simulink model "Copy_of_fast_powertrain"  (R2020b)
settings: Solver=FixedStepAuto  StartTime=0  StopTime=t(end)  RelTol=1e-3
PreLoadFcn:
  | C_sc = 1;
StartFcn:
  | C_sc = 1;
values from neighbouring files (symbols this model uses):
  fc_power_array = [900 900 900 900 900 900 900 900 900 900 900 900 ... (24566 elements, 71x346)]    [fc_power_climb_dp.mat]    (also in fc_power_cruise_dp.mat = [0 0 0 0 0 0 0 0 0 0 0 0 ... (32589 elements, 71x459)]; fc_power_descend_dp.mat = [285.411057245 285.411057245 285.411057245 285.411057245 285; fc_power_takeoff_dp.mat = [0 0 0 0 0 0 0 0 0 0 0 0 ... (23714 elements, 71x334)])
  Ts = old_data.Ts    [model_fc.m]
undefined symbols (not defined in the file or in its folder): DiscIntNeverNeededParam, Ion, Lithium, w
libraries: neural x50, powerlib x30, fuzblock x7, electricdrivelib x2, lib_converters x2, simulink x1
(part 3 of 5)

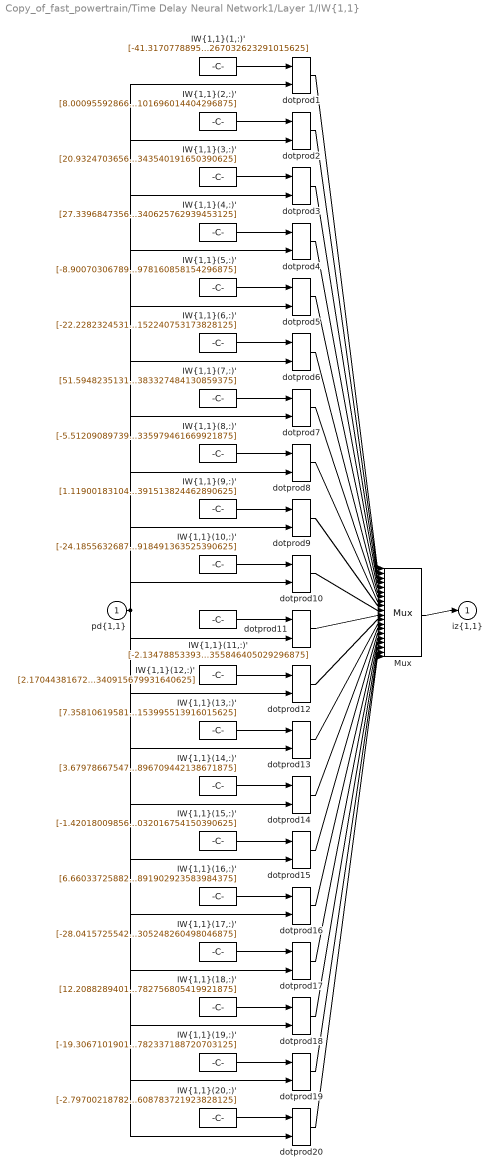
== system Copy_of_fast_powertrain/Time Delay Neural Network1/Layer 1/IW{1,1} ==
  "pd{1,1}" : Inport  PortDimensions=20  SampleTime=0.01
      mask Display: e = 0.06;c1 = [120 230 180]/255;c2 = ([120 230 180]+0)/(256+128);c3 = ([120 230 180]+128)/(256+128);patch([0 1 1 0],[0 0 1 1],c1);patch([0 1 1 1-e 1-e 0+e],[0 0 1 1-e 0+e 0+e],c2);patch([0 0 1 1-e 0+e 0+e],[0 1 1 1-e 1-e 0+e],c3);plot([0 1 1 0 0],[0 0 1 1 0]);
  "IW{1,1}(1,:)'" : Constant  Value=[-41.3170778895787549345186562277376651763916015625;-24.0887056388310867305335705168545246124267578125;-13.8798772268015415676245538634248077869415283203125;-11.567409242390937151867547072470188140869140625;-7.356579925855793788969094748608767986297607421875;4.9515916542348659135086563765071332454681396484375;14.3524439434296144924019245081581175327301025390625;16.54972712574036819432876654900610446929931640625;14.0243285040616729730800216202624142169952392578125;8.05588338287137872839593910612165927886962890625;0.244736738010354282213398846579366363584995269775390625;-6.6453737162459614040699307224713265895843505859375;-8.08441524115644227777011110447347164154052734375;-3.094343005952360226018527100677601993083953857421875;4.26970438586587075491252107894979417324066162109375;3.5510471509297900638557621277868747711181640625;1.931204814168190342371644874219782650470733642578125;5.147881514928489110616283142007887363433837890625;15.346019511090471354464170872233808040618896484375;28.89157804877809354593409807421267032623291015625]
      mask Display: e = 0.06;c1 = [120 150 230]/255;c2 = ([120 150 230]+0)/383;c3 = ([120 150 230]+128)/383;patch([0 1 1 0],[0 0 1 1],c1);patch([0 1 1 1-e 1-e 0+e],[0 0 1 1-e 0+e 0+e],c2);patch([0 0 1 1-e 0+e 0+e],[0 1 1 1-e 1-e 0+e],c3);plot([0 1 1 0 0],[0 0 1 1 0]);disp('Weights');
  "IW{1,1}(10,:)'" : Constant  Value=[-24.185563268711344875327995396219193935394287109375;-17.05035411347990503827531938441097736358642578125;-13.6433375683293132141216119634918868541717529296875;-10.6339863508851077966710363398306071758270263671875;-8.167743630631310480794127215631306171417236328125;-7.68393810138619404170867710490711033344268798828125;-7.310595578676071681911707855761051177978515625;-6.6070230562044311994895906536839902400970458984375;-4.7908556067367129571721307002007961273193359375;-2.130885890521920345008766162209212779998779296875;0.6736905781048412311662332285777665674686431884765625;3.79217370987275526061921482323668897151947021484375;4.9231950163727358216192442341707646846771240234375;6.56156027024927990254354881471954286098480224609375;5.07963430191251763545778885600157082080841064453125;4.58522380417822095211022315197624266147613525390625;4.63238649648575506745373786543495953083038330078125;8.33057908449168138531604199670255184173583984375;16.600928369549830421192382345907390117645263671875;29.7591641296045281706028617918491363525390625]
      mask Display: e = 0.06;c1 = [120 150 230]/255;c2 = ([120 150 230]+0)/383;c3 = ([120 150 230]+128)/383;patch([0 1 1 0],[0 0 1 1],c1);patch([0 1 1 1-e 1-e 0+e],[0 0 1 1-e 0+e 0+e],c2);patch([0 0 1 1-e 0+e 0+e],[0 1 1 1-e 1-e 0+e],c3);plot([0 1 1 0 0],[0 0 1 1 0]);disp('Weights');
  "IW{1,1}(11,:)'" : Constant  Value=[-2.1347885339333476650836018961854279041290283203125;19.6289364994059951641247607767581939697265625;4.14715056300510287456972946529276669025421142578125;1.261358625362304142214497915119864046573638916015625;3.84623883470571126252934845979325473308563232421875;-7.1682582085659962700674441293813288211822509765625;-3.736923646637921425650574747123755514621734619140625;-5.88069141749093748927634806022979319095611572265625;-5.55573602274217481777895955019630491733551025390625;4.31752698833330317285117416759021580219268798828125;-1.1252300459187354331191954770474694669246673583984375;4.05713927249998551616272379760630428791046142578125;1.197702286576397767703383578918874263763427734375;-1.9553589340063435297878413621219806373119354248046875;1.6492618632624937990982516566873528063297271728515625;0.2910930951259309562573207585955969989299774169921875;-7.48533898139895992329684304422698915004730224609375;-5.0718983260841241644811816513538360595703125;-9.951981369443966940480095217935740947723388671875;16.351487277274980414176752674393355846405029296875]
      mask Display: e = 0.06;c1 = [120 150 230]/255;c2 = ([120 150 230]+0)/383;c3 = ([120 150 230]+128)/383;patch([0 1 1 0],[0 0 1 1],c1);patch([0 1 1 1-e 1-e 0+e],[0 0 1 1-e 0+e 0+e],c2);patch([0 0 1 1-e 0+e 0+e],[0 1 1 1-e 1-e 0+e],c3);plot([0 1 1 0 0],[0 0 1 1 0]);disp('Weights');
  "IW{1,1}(12,:)'" : Constant  Value=[2.170443816728891750500451962579973042011260986328125;4.831373528298119168766788789071142673492431640625;3.720585501332140498931266847648657858371734619140625;-0.318133659340753049971084465141757391393184661865234375;-0.475728325064818824419177190065965987741947174072265625;-1.51040958520863544123358224169351160526275634765625;2.69378750685471768377965418039821088314056396484375;-1.96104009447486671291471793665550649166107177734375;-3.015653540352828176906996304751373827457427978515625;0.29681634914598553631748245607013814151287078857421875;-3.39010087809587101759234428755007684230804443359375;-3.109983657771648868362035500467754900455474853515625;-2.5953120035258248066156738786958158016204833984375;2.638838351776431334627659452962689101696014404296875;5.737602587752082428096400690264999866485595703125;2.73716197207968914284492711885832250118255615234375;-1.03884155019751123205651310854591429233551025390625;0.70165190413190947626986826435313560068607330322265625;-6.92628258625202430920353435794822871685028076171875;-5.28110531151323758791704676696099340915679931640625]
      mask Display: e = 0.06;c1 = [120 150 230]/255;c2 = ([120 150 230]+0)/383;c3 = ([120 150 230]+128)/383;patch([0 1 1 0],[0 0 1 1],c1);patch([0 1 1 1-e 1-e 0+e],[0 0 1 1-e 0+e 0+e],c2);patch([0 0 1 1-e 0+e 0+e],[0 1 1 1-e 1-e 0+e],c3);plot([0 1 1 0 0],[0 0 1 1 0]);disp('Weights');
  "IW{1,1}(13,:)'" : Constant  Value=[7.358106195812315064586073276586830615997314453125;1.6831218618925074537173713906668126583099365234375;-2.8683861634367673332235426642000675201416015625;-3.85951595603854524796361147309653460979461669921875;-2.419423126387662659197985703940503299236297607421875;-1.588508626987817251574597321450710296630859375;-1.37264008448260010908370531979016959667205810546875;-1.54854636023814773437834446667693555355072021484375;-0.10374636418391712522346637115333578549325466156005859375;-0.5967477756502417296502471799612976610660552978515625;0.43226922179724536210443375239265151321887969970703125;0.5628800436407732643573353925603441894054412841796875;0.8431480665077806246898717290605418384075164794921875;0.63425152767940617959396831793128512799739837646484375;1.3560400000311558788013144294382072985172271728515625;1.06751403398893529583801864646375179290771484375;-1.1827681419481888003275571463746018707752227783203125;-4.5508660633518918103845862788148224353790283203125;-8.1547629852644458736676824628375470638275146484375;-12.0765016778454796764208367676474153995513916015625]
      mask Display: e = 0.06;c1 = [120 150 230]/255;c2 = ([120 150 230]+0)/383;c3 = ([120 150 230]+128)/383;patch([0 1 1 0],[0 0 1 1],c1);patch([0 1 1 1-e 1-e 0+e],[0 0 1 1-e 0+e 0+e],c2);patch([0 0 1 1-e 0+e 0+e],[0 1 1 1-e 1-e 0+e],c3);plot([0 1 1 0 0],[0 0 1 1 0]);disp('Weights');
  "IW{1,1}(14,:)'" : Constant  Value=[3.67978667547009674620994701399467885494232177734375;-2.22690009056678572818555039702914655208587646484375;-0.79222376523893933697451075204298831522464752197265625;-6.8093908520768895442643042770214378833770751953125;-2.572056436179115390672222929424606263637542724609375;-1.0626538149219673101697480888105928897857666015625;0.5276216253397276734204979220521636307239532470703125;2.0319562855862702832610011682845652103424072265625;4.9281641317842979077568088541738688945770263671875;2.773369998445488260330193952540867030620574951171875;0.96562902640608372362152067580609582364559173583984375;6.66870819884032695057385353720746934413909912109375;4.0853706891057530725674951099790632724761962890625;-3.780792512882989786504595031146891415119171142578125;-7.9357944400793751782430263119749724864959716796875;-6.37633154443981009507069757091812789440155029296875;0.75252557231104411084032790313358418643474578857421875;3.713808685864766090389821329154074192047119140625;3.38778820457910878616303307353518903255462646484375;4.62408844976101374157906320760957896709442138671875]
      mask Display: e = 0.06;c1 = [120 150 230]/255;c2 = ([120 150 230]+0)/383;c3 = ([120 150 230]+128)/383;patch([0 1 1 0],[0 0 1 1],c1);patch([0 1 1 1-e 1-e 0+e],[0 0 1 1-e 0+e 0+e],c2);patch([0 0 1 1-e 0+e 0+e],[0 1 1 1-e 1-e 0+e],c3);plot([0 1 1 0 0],[0 0 1 1 0]);disp('Weights');
  "IW{1,1}(15,:)'" : Constant  Value=[-1.420180098569664206564766573137603700160980224609375;-5.51110982430032692036547814495861530303955078125;-5.20947745625726010842981850146315991878509521484375;-14.6997746442128800481441430747509002685546875;-8.8563278920764787471853196620941162109375;-0.9626373423566885190183484155568294227123260498046875;6.19541237091466800990247065783478319644927978515625;8.8144073732205558968644254491664469242095947265625;12.296059111145755338156959624029695987701416015625;7.9205582139870909230694451252929866313934326171875;3.785811551668564423067664392874576151371002197265625;-5.5243128402192116510605046642012894153594970703125;-10.001006466530355965005583129823207855224609375;-8.889928686249508160699406289495527744293212890625;-3.84096755903057474057504805386997759342193603515625;2.4065504070994290231055856565944850444793701171875;3.914269531419424907880966202355921268463134765625;6.43574838587781972165657862205989658832550048828125;20.02672266276139367846553795970976352691650390625;-8.6135092808080031545614474453032016754150390625]
      mask Display: e = 0.06;c1 = [120 150 230]/255;c2 = ([120 150 230]+0)/383;c3 = ([120 150 230]+128)/383;patch([0 1 1 0],[0 0 1 1],c1);patch([0 1 1 1-e 1-e 0+e],[0 0 1 1-e 0+e 0+e],c2);patch([0 0 1 1-e 0+e 0+e],[0 1 1 1-e 1-e 0+e],c3);plot([0 1 1 0 0],[0 0 1 1 0]);disp('Weights');
  "IW{1,1}(16,:)'" : Constant  Value=[6.6603372588299354362106896587647497653961181640625;-0.8908372930182395510456672127475030720233917236328125;5.327501255420738601742414175532758235931396484375;15.32497122996134208960938849486410617828369140625;10.790263493254013127398138749413192272186279296875;1.0196787390633499370551362517289817333221435546875;-5.69550501395408392824037946411408483982086181640625;-11.3091877191841962968510415521450340747833251953125;-10.578463028595951556098953005857765674591064453125;-9.5307296775407497335663720150478184223175048828125;-2.19973343032226242854676456772722303867340087890625;3.735648738789860257014652233920060098171234130859375;11.079809353653434556008505751378834247589111328125;8.9052404932124584746588880079798400402069091796875;3.4040744108171434589849013718776404857635498046875;-1.225929473324251173238508272334001958370208740234375;-3.28411757385438018985723829246126115322113037109375;-10.3218805156491679753116841311566531658172607421875;-12.8732991153864446687293821014463901519775390625;3.45410954567542116677714147954247891902923583984375]
      mask Display: e = 0.06;c1 = [120 150 230]/255;c2 = ([120 150 230]+0)/383;c3 = ([120 150 230]+128)/383;patch([0 1 1 0],[0 0 1 1],c1);patch([0 1 1 1-e 1-e 0+e],[0 0 1 1-e 0+e 0+e],c2);patch([0 0 1 1-e 0+e 0+e],[0 1 1 1-e 1-e 0+e],c3);plot([0 1 1 0 0],[0 0 1 1 0]);disp('Weights');
  "IW{1,1}(17,:)'" : Constant  Value=[-28.04157255425118222547098412178456783294677734375;-5.3809637724850656326225362136028707027435302734375;5.17695541887508081657642833306454122066497802734375;11.16804148725753975668339990079402923583984375;12.0601664903482248547561539453454315662384033203125;7.36291293894431664313060537097044289112091064453125;5.5119750429278298042845563031733036041259765625;-2.661671141807496088205198248033411800861358642578125;-4.4897286315137865386759585817344486713409423828125;-0.502920581020447343689738772809505462646484375;-0.5422578739548782333912413378129713237285614013671875;-1.716441764453623619601785321719944477081298828125;1.1676228984111858277827877827803604304790496826171875;5.550100097403696253195448662154376506805419921875;7.51119188051158293006892563425935804843902587890625;5.740538523639262535880334326066076755523681640625;1.8215987865340081963694274236331693828105926513671875;-3.41564694209144281700218925834633409976959228515625;-2.506787719899347788299337480566464364528656005859375;-10.8136694568940452398919660481624305248260498046875]
      mask Display: e = 0.06;c1 = [120 150 230]/255;c2 = ([120 150 230]+0)/383;c3 = ([120 150 230]+128)/383;patch([0 1 1 0],[0 0 1 1],c1);patch([0 1 1 1-e 1-e 0+e],[0 0 1 1-e 0+e 0+e],c2);patch([0 0 1 1-e 0+e 0+e],[0 1 1 1-e 1-e 0+e],c3);plot([0 1 1 0 0],[0 0 1 1 0]);disp('Weights');
  "IW{1,1}(18,:)'" : Constant  Value=[12.2088289401585239346559319528751075267791748046875;11.207627170941886873833936988376080989837646484375;8.120166375458776286677675670944154262542724609375;4.45666694105473037978981665219180285930633544921875;-4.4224351247064124237340365652926266193389892578125;-6.20601126716516926506983509170822799205780029296875;-1.9195754434346776751141305794590152800083160400390625;-3.13496102854807379145540835452266037464141845703125;-2.32668178326190489002556205377914011478424072265625;0.670511817366107987226087061571888625621795654296875;0.89232140437771600982586051031830720603466033935546875;0.55752894691838772445180438808165490627288818359375;-3.33344947856499818072961716097779572010040283203125;1.8208920236868164632682010051212273538112640380859375;5.4889024169390694396497565321624279022216796875;1.5847163583448542478748777284636162221431732177734375;-5.3921423981682092829714747495017945766448974609375;-8.405302129591763815597005304880440235137939453125;-8.864741878767407712302883737720549106597900390625;-3.543055787799016087546988273970782756805419921875]
      mask Display: e = 0.06;c1 = [120 150 230]/255;c2 = ([120 150 230]+0)/383;c3 = ([120 150 230]+128)/383;patch([0 1 1 0],[0 0 1 1],c1);patch([0 1 1 1-e 1-e 0+e],[0 0 1 1-e 0+e 0+e],c2);patch([0 0 1 1-e 0+e 0+e],[0 1 1 1-e 1-e 0+e],c3);plot([0 1 1 0 0],[0 0 1 1 0]);disp('Weights');
  "IW{1,1}(19,:)'" : Constant  Value=[-19.30671019010623012945870868861675262451171875;-21.983671689361745649193835561163723468780517578125;-11.103043353793257352890577749349176883697509765625;-0.279565088451577903327915919362567365169525146484375;9.0057348671534942496919029508717358112335205078125;11.408177187217649617423376184888184070587158203125;10.029518245539403409338774508796632289886474609375;4.33827750612211815450791618786752223968505859375;6.97972260717902681648183715878985822200775146484375;8.3558582696726748650917215854860842227935791015625;3.49812962932533455528982813120819628238677978515625;1.094973913609437854432826497941277921199798583984375;0.82543490581334777456135043394169770181179046630859375;-0.68629990853895694868924692855216562747955322265625;0.0468479576123603524973049161417293362319469451904296875;-4.7912054993083206255732875433750450611114501953125;-1.786395953938544334249627354438416659832000732421875;-6.22266231890149068561868261895142495632171630859375;6.907932831061526002258688095025718212127685546875;5.413336757037843227635676157660782337188720703125]
      mask Display: e = 0.06;c1 = [120 150 230]/255;c2 = ([120 150 230]+0)/383;c3 = ([120 150 230]+128)/383;patch([0 1 1 0],[0 0 1 1],c1);patch([0 1 1 1-e 1-e 0+e],[0 0 1 1-e 0+e 0+e],c2);patch([0 0 1 1-e 0+e 0+e],[0 1 1 1-e 1-e 0+e],c3);plot([0 1 1 0 0],[0 0 1 1 0]);disp('Weights');
  "IW{1,1}(2,:)'" : Constant  Value=[8.0009559286644194031623555929400026798248291015625;0.29799913640694886129978158351150341331958770751953125;2.199307294349767349928015391924418509006500244140625;-0.101158104774415169568868577698594890534877777099609375;-3.272729845188205644035406294278800487518310546875;2.52183259058507047711827908642590045928955078125;-1.46306994719022664952490231371484696865081787109375;-0.571724712775646626283787554712034761905670166015625;0.4244111816213844701195512243430130183696746826171875;-2.11138170909325406654488688218407332897186279296875;-0.1092852808671377629057275271406979300081729888916015625;-7.0818638804236986317164337378926575183868408203125;-1.57683215732416659449199869413860142230987548828125;3.46336741857540975075835376628674566745758056640625;4.80213581541669309871167570236138999462127685546875;2.82902758629478956464708971907384693622589111328125;-1.7424597394520520143856856520869769155979156494140625;-3.902954257014578320905684449826367199420928955078125;2.9544813906346103493660848471336066722869873046875;-9.4713163438792360437901152181439101696014404296875]
      mask Display: e = 0.06;c1 = [120 150 230]/255;c2 = ([120 150 230]+0)/383;c3 = ([120 150 230]+128)/383;patch([0 1 1 0],[0 0 1 1],c1);patch([0 1 1 1-e 1-e 0+e],[0 0 1 1-e 0+e 0+e],c2);patch([0 0 1 1-e 0+e 0+e],[0 1 1 1-e 1-e 0+e],c3);plot([0 1 1 0 0],[0 0 1 1 0]);disp('Weights');
  "IW{1,1}(20,:)'" : Constant  Value=[-2.797002187821615137863773270510137081146240234375;-10.31295322399305547378389746882021427154541015625;-1.55660953829066528442126582376658916473388671875;3.35580071000512081269562258967198431491851806640625;5.9643923538503411663214137661270797252655029296875;5.39805766669024933435139246284961700439453125;2.014178251230946958827416892745532095432281494140625;-0.5077485053936430237087051864364184439182281494140625;0.44283688715125801849126219167374074459075927734375;-0.84923676595938868416624245583079755306243896484375;-1.0839363293868820026233379394398070871829986572265625;2.74830351179496457092454875237308442592620849609375;5.96715115443901300551488020573742687702178955078125;10.446421954846481838785621221177279949188232421875;9.2391410777889628747061578906141221523284912109375;3.9956120733058124727676840848289430141448974609375;-2.73014654632758801966474493383429944515228271484375;-4.92810777807717403931064836797304451465606689453125;-6.188792555902221437236221390776336193084716796875;-14.4144108890875362050110197742469608783721923828125]
      mask Display: e = 0.06;c1 = [120 150 230]/255;c2 = ([120 150 230]+0)/383;c3 = ([120 150 230]+128)/383;patch([0 1 1 0],[0 0 1 1],c1);patch([0 1 1 1-e 1-e 0+e],[0 0 1 1-e 0+e 0+e],c2);patch([0 0 1 1-e 0+e 0+e],[0 1 1 1-e 1-e 0+e],c3);plot([0 1 1 0 0],[0 0 1 1 0]);disp('Weights');
  "IW{1,1}(3,:)'" : Constant  Value=[20.932470365689123781294256332330405712127685546875;18.254007786078663144735401147045195102691650390625;11.545421494161882236539895529858767986297607421875;-0.4887756653028054731890961193130351603031158447265625;-8.76398413124098851767485029995441436767578125;-12.57365231422826212792642763815820217132568359375;-7.46222359613562158386912415153346955776214599609375;-4.808412478315300830900014261715114116668701171875;-6.0961149428762926305580549524165689945220947265625;-7.3019081107598680091541609726846218109130859375;-3.070212599719938761921866898774169385433197021484375;-1.3184986949957842039538036260637454688549041748046875;-1.2993064234001974188714711999637074768543243408203125;0.406971975746562630860125864273868501186370849609375;-1.0449934646656526826546951269847340881824493408203125;6.169523300947691524243055027909576892852783203125;1.81080629847727525572054219082929193973541259765625;5.59354256645015102122897587832994759082794189453125;-1.485107007839122861270197972771711647510528564453125;-10.7319771586214418590543573372997343540191650390625]
      mask Display: e = 0.06;c1 = [120 150 230]/255;c2 = ([120 150 230]+0)/383;c3 = ([120 150 230]+128)/383;patch([0 1 1 0],[0 0 1 1],c1);patch([0 1 1 1-e 1-e 0+e],[0 0 1 1-e 0+e 0+e],c2);patch([0 0 1 1-e 0+e 0+e],[0 1 1 1-e 1-e 0+e],c3);plot([0 1 1 0 0],[0 0 1 1 0]);disp('Weights');
  "IW{1,1}(4,:)'" : Constant  Value=[27.339684735619670163941918872296810150146484375;8.496357856765598626225255429744720458984375;-6.362755084862403265333341551013290882110595703125;-12.7773678444801674913833267055451869964599609375;-10.492634466608620869010337628424167633056640625;-9.67105286856625667724074446596205234527587890625;-3.440768679224401438432323629967868328094482421875;0.2963145832070235297095450732740573585033416748046875;5.7437713069473463889380582259036600589752197265625;0.3476258632510009771721115612308494746685028076171875;0.552428702577281161012479060445912182331085205078125;3.393992684218976929599875802523456513881683349609375;-1.6843270831895862382765471920720301568508148193359375;-6.6691540021836797080823089345358312129974365234375;-7.6569929153395168697215922293253242969512939453125;-4.88877927553946367567050401703454554080963134765625;-0.78681722837249612467758197453804314136505126953125;-0.0568690636677235961116139151272363960742950439453125;6.4993261608193648726228275336325168609619140625;8.56317161450824215762622770853340625762939453125]
      mask Display: e = 0.06;c1 = [120 150 230]/255;c2 = ([120 150 230]+0)/383;c3 = ([120 150 230]+128)/383;patch([0 1 1 0],[0 0 1 1],c1);patch([0 1 1 1-e 1-e 0+e],[0 0 1 1-e 0+e 0+e],c2);patch([0 0 1 1-e 0+e 0+e],[0 1 1 1-e 1-e 0+e],c3);plot([0 1 1 0 0],[0 0 1 1 0]);disp('Weights');
  "IW{1,1}(5,:)'" : Constant  Value=[-8.9007030678935148415575895342044532299041748046875;9.4651280143608769179763839929364621639251708984375;2.459275957901349674017410507076419889926910400390625;3.7583207043845927586289690225385129451751708984375;1.82154654944120775184046578942798078060150146484375;1.421627956337805809283736380166374146938323974609375;-0.7058342521599818564226325179333798587322235107421875;-2.992863439742887265992976608686149120330810546875;-5.2068906654741358153160035726614296436309814453125;-1.66773704253629428961858138791285455226898193359375;-1.9184820671787401469288170119398273527622222900390625;-5.189770753495704269653288065455853939056396484375;-3.424954548731278247686304894159547984600067138671875;3.79075968895624715315761932288296520709991455078125;7.4365298630443561478386982344090938568115234375;6.32941151198017326606759525020606815814971923828125;-1.2726758449697410657819318657857365906238555908203125;-5.25567297078029493917483705445192754268646240234375;-2.26274858455408978130662944749929010868072509765625;-4.2604163572358100253723023342899978160858154296875]
      mask Display: e = 0.06;c1 = [120 150 230]/255;c2 = ([120 150 230]+0)/383;c3 = ([120 150 230]+128)/383;patch([0 1 1 0],[0 0 1 1],c1);patch([0 1 1 1-e 1-e 0+e],[0 0 1 1-e 0+e 0+e],c2);patch([0 0 1 1-e 0+e 0+e],[0 1 1 1-e 1-e 0+e],c3);plot([0 1 1 0 0],[0 0 1 1 0]);disp('Weights');
  "IW{1,1}(6,:)'" : Constant  Value=[-22.22823245318267026959802024066448211669921875;-2.61267557073272627121696132235229015350341796875;-6.09690996180808664206551839015446603298187255859375;0.5252305434929851468695005678455345332622528076171875;5.18797140766390985078260200680233538150787353515625;1.020876156381517407822911991388536989688873291015625;8.70257213333764667595460196025669574737548828125;5.2204624128180956432743187178857624530792236328125;-0.8366628262687212380654955268255434930324554443359375;-0.373197414506467595174399320967495441436767578125;-6.92678541912431366966984569444321095943450927734375;0.10324869827143635936383958551232353784143924713134765625;1.2418435739121991279176882017054595053195953369140625;1.0557948454136596438956985366530716419219970703125;3.01402759675961018359657828113995492458343505859375;4.22146805757340981557490522391162812709808349609375;7.247146300064496671211600187234580516815185546875;4.3041061071129007586932857520878314971923828125;-9.6874140400343602408383958390913903713226318359375;-3.2759926367543688030536941369064152240753173828125]
      mask Display: e = 0.06;c1 = [120 150 230]/255;c2 = ([120 150 230]+0)/383;c3 = ([120 150 230]+128)/383;patch([0 1 1 0],[0 0 1 1],c1);patch([0 1 1 1-e 1-e 0+e],[0 0 1 1-e 0+e 0+e],c2);patch([0 0 1 1-e 0+e 0+e],[0 1 1 1-e 1-e 0+e],c3);plot([0 1 1 0 0],[0 0 1 1 0]);disp('Weights');
  "IW{1,1}(7,:)'" : Constant  Value=[51.5948235131668724307019147090613842010498046875;18.479203641606357422233486431650817394256591796875;-0.1138401529098100883885535949957557022571563720703125;-6.98963796653444280337907912326045334339141845703125;-11.170389097549676904463922255672514438629150390625;-10.4819913877186223771786899305880069732666015625;-9.247598137383402416844546678476035594940185546875;-7.17700869258198981270879812655039131641387939453125;-2.6320741480940785805842097033746540546417236328125;-2.602296546208933580857092238147743046283721923828125;0.2042727877142753722949919392704032361507415771484375;3.9466909235221550034111714921891689300537109375;2.978154313847202416809523128904402256011962890625;-0.2970520106042477959107372953440062701702117919921875;-4.93554185989632543396510300226509571075439453125;-8.604976836124681227602195576764643192291259765625;-8.068677822123898835116051486693322658538818359375;-8.78376927972495735730262822471559047698974609375;0.47388675040789696168985756230540573596954345703125;16.67770704955804461633306345902383327484130859375]
      mask Display: e = 0.06;c1 = [120 150 230]/255;c2 = ([120 150 230]+0)/383;c3 = ([120 150 230]+128)/383;patch([0 1 1 0],[0 0 1 1],c1);patch([0 1 1 1-e 1-e 0+e],[0 0 1 1-e 0+e 0+e],c2);patch([0 0 1 1-e 0+e 0+e],[0 1 1 1-e 1-e 0+e],c3);plot([0 1 1 0 0],[0 0 1 1 0]);disp('Weights');
  "IW{1,1}(8,:)'" : Constant  Value=[-5.5120908973902178473736057640053331851959228515625;-0.08857216638173925904453653856762684881687164306640625;-6.8524858480580181918639937066473066806793212890625;-4.2453872729833204147098513203673064708709716796875;-1.7177497627532272161943183164112269878387451171875;4.06465131407648794237275069463066756725311279296875;5.13777173224305361287633786560036242008209228515625;3.56461861949192293508303919224999845027923583984375;-0.453789369166626543883324984562932513654232025146484375;-0.56670916479507804641713164528482593595981597900390625;-4.24873351646846497686738075572066009044647216796875;2.640255431642579697637529534404166042804718017578125;-1.24500832619264745204645805642940104007720947265625;1.492862977137506153013646326144225895404815673828125;1.0004088100251049553435223060660064220428466796875;2.33866054122455846453476624446921050548553466796875;5.0613013830595861008987412787973880767822265625;3.733246583413986297017572724143974483013153076171875;-5.1544106155657498646860403823666274547576904296875;-4.80560696182090918426865755463950335979461669921875]
      mask Display: e = 0.06;c1 = [120 150 230]/255;c2 = ([120 150 230]+0)/383;c3 = ([120 150 230]+128)/383;patch([0 1 1 0],[0 0 1 1],c1);patch([0 1 1 1-e 1-e 0+e],[0 0 1 1-e 0+e 0+e],c2);patch([0 0 1 1-e 0+e 0+e],[0 1 1 1-e 1-e 0+e],c3);plot([0 1 1 0 0],[0 0 1 1 0]);disp('Weights');
  "IW{1,1}(9,:)'" : Constant  Value=[1.1190018310491545161511339756543748080730438232421875;-9.99456168542398160070661106146872043609619140625;-6.05258353940696025574652594514191150665283203125;-7.28848460783531582052319208742119371891021728515625;-0.8187356429915058075863498743274249136447906494140625;5.16051913868130096574304843670688569545745849609375;5.9688291019320995900443449500016868114471435546875;2.700108935388829234369723053532652556896209716796875;2.77621122768115125012400312698446214199066162109375;-1.219439809609997649175738843041472136974334716796875;-0.65899091759310446381192605258547700941562652587890625;-2.929613833743692108413370078778825700283050537109375;0.1052108163845257848834080505184829235076904296875;-0.34501059064822758859492068950203247368335723876953125;1.1175172915267108653125660566729493439197540283203125;4.27864428805897745178299373947083950042724609375;5.42493416790487259504516259767115116119384765625;2.13665947942197487208204620401374995708465576171875;-0.259858993996790577085675977286882698535919189453125;-7.78855454396885082957169288420118391513824462890625]
      mask Display: e = 0.06;c1 = [120 150 230]/255;c2 = ([120 150 230]+0)/383;c3 = ([120 150 230]+128)/383;patch([0 1 1 0],[0 0 1 1],c1);patch([0 1 1 1-e 1-e 0+e],[0 0 1 1-e 0+e 0+e],c2);patch([0 0 1 1-e 0+e 0+e],[0 1 1 1-e 1-e 0+e],c3);plot([0 1 1 0 0],[0 0 1 1 0]);disp('Weights');
  Mux : Mux  Inputs=20
      mask Display: e = 0.06;c1 = [120 150 230]/255;c2 = ([120 150 230]+0)/383;c3 = ([120 150 230]+128)/383;patch([0 1 1 0],[0 0 1 1],c1);patch([0 1 1 1-e 1-e 0+e],[0 0 1 1-e 0+e 0+e],c2);patch([0 0 1 1-e 0+e 0+e],[0 1 1 1-e 1-e 0+e],c3);plot([0 1 1 0 0],[0 0 1 1 0]);disp('Mux');
  dotprod{1..20} (20 alike) : neural/Weight Functions/dotprod
  "iz{1,1}" : Outport
      mask Display: e = 0.06;c1 = [120 230 180]/255;c2 = ([120 230 180]+0)/(256+128);c3 = ([120 230 180]+128)/(256+128);patch([0 1 1 0],[0 0 1 1],c1);patch([0 1 1 1-e 1-e 0+e],[0 0 1 1-e 0+e 0+e],c2);patch([0 0 1 1-e 0+e 0+e],[0 1 1 1-e 1-e 0+e],c3);plot([0 1 1 0 0],[0 0 1 1 0]);
  wires:
  Mux/1 -> "iz{1,1}"/1
  dotprod20/1 -> Mux/20
  "IW{1,1}(20,:)'"/1 -> dotprod20/1
  dotprod19/1 -> Mux/19
  "IW{1,1}(19,:)'"/1 -> dotprod19/1
  dotprod18/1 -> Mux/18
  "IW{1,1}(18,:)'"/1 -> dotprod18/1
  dotprod17/1 -> Mux/17
  "IW{1,1}(17,:)'"/1 -> dotprod17/1
  dotprod16/1 -> Mux/16
  "IW{1,1}(16,:)'"/1 -> dotprod16/1
  dotprod15/1 -> Mux/15
  "IW{1,1}(15,:)'"/1 -> dotprod15/1
  dotprod14/1 -> Mux/14
  "IW{1,1}(14,:)'"/1 -> dotprod14/1
  dotprod13/1 -> Mux/13
  "IW{1,1}(13,:)'"/1 -> dotprod13/1
  dotprod12/1 -> Mux/12
  "IW{1,1}(12,:)'"/1 -> dotprod12/1
  dotprod11/1 -> Mux/11
  "IW{1,1}(11,:)'"/1 -> dotprod11/1
  dotprod10/1 -> Mux/10
  "IW{1,1}(10,:)'"/1 -> dotprod10/1
  dotprod9/1 -> Mux/9
  "IW{1,1}(9,:)'"/1 -> dotprod9/1
  dotprod8/1 -> Mux/8
  "IW{1,1}(8,:)'"/1 -> dotprod8/1
  dotprod7/1 -> Mux/7
  "IW{1,1}(7,:)'"/1 -> dotprod7/1
  dotprod6/1 -> Mux/6
  "IW{1,1}(6,:)'"/1 -> dotprod6/1
  dotprod5/1 -> Mux/5
  "IW{1,1}(5,:)'"/1 -> dotprod5/1
  dotprod4/1 -> Mux/4
  "IW{1,1}(4,:)'"/1 -> dotprod4/1
  dotprod3/1 -> Mux/3
  "IW{1,1}(3,:)'"/1 -> dotprod3/1
  dotprod2/1 -> Mux/2
  "IW{1,1}(2,:)'"/1 -> dotprod2/1
  dotprod1/1 -> Mux/1
  "pd{1,1}"/1 -> dotprod20/2, dotprod19/2, dotprod18/2, dotprod17/2, dotprod16/2, dotprod15/2, dotprod14/2, dotprod13/2, dotprod12/2, dotprod11/2, dotprod10/2, dotprod9/2, dotprod8/2, dotprod7/2, dotprod6/2, dotprod5/2, dotprod4/2, dotprod3/2, dotprod2/2, dotprod1/2
  "IW{1,1}(1,:)'"/1 -> dotprod1/1

== system Copy_of_fast_powertrain/Time Delay Neural Network1/Layer 2/Delays 1 ==
  "p{2}" : Inport  PortDimensions=20  SampleTime=0.01
      mask Display: e = 0.06;c1 = [120 230 180]/255;c2 = ([120 230 180]+0)/(256+128);c3 = ([120 230 180]+128)/(256+128);patch([0 1 1 0],[0 0 1 1],c1);patch([0 1 1 1-e 1-e 0+e],[0 0 1 1-e 0+e 0+e],c2);patch([0 0 1 1-e 0+e 0+e],[0 1 1 1-e 1-e 0+e],c3);plot([0 1 1 0 0],[0 0 1 1 0]);
  mux : Mux  Inputs=1
      mask Display: e = 0.06;c1 = [120 150 230]/255;c2 = ([120 150 230]+0)/383;c3 = ([120 150 230]+128)/383;patch([0 1 1 0],[0 0 1 1],c1);patch([0 1 1 1-e 1-e 0+e],[0 0 1 1-e 0+e 0+e],c2);patch([0 0 1 1-e 0+e 0+e],[0 1 1 1-e 1-e 0+e],c3);plot([0 1 1 0 0],[0 0 1 1 0]);disp('Mux')
  "pd{2,1}" : Outport
      mask Display: e = 0.06;c1 = [120 230 180]/255;c2 = ([120 230 180]+0)/(256+128);c3 = ([120 230 180]+128)/(256+128);patch([0 1 1 0],[0 0 1 1],c1);patch([0 1 1 1-e 1-e 0+e],[0 0 1 1-e 0+e 0+e],c2);patch([0 0 1 1-e 0+e 0+e],[0 1 1 1-e 1-e 0+e],c3);plot([0 1 1 0 0],[0 0 1 1 0]);
  wires:
  mux/1 -> "pd{2,1}"/1
  "p{2}"/1 -> mux/1

== system Copy_of_fast_powertrain/Time Delay Neural Network1/Layer 2/LW{2,1} ==
  "ad{2,1}" : Inport  PortDimensions=20  SampleTime=0.01
      mask Display: e = 0.06;c1 = [120 230 180]/255;c2 = ([120 230 180]+0)/(256+128);c3 = ([120 230 180]+128)/(256+128);patch([0 1 1 0],[0 0 1 1],c1);patch([0 1 1 1-e 1-e 0+e],[0 0 1 1-e 0+e 0+e],c2);patch([0 0 1 1-e 0+e 0+e],[0 1 1 1-e 1-e 0+e],c3);plot([0 1 1 0 0],[0 0 1 1 0]);
  "IW{2,1}(1,:)'" : Constant  Value=[0.8146129313273871019873695331625640392303466796875;-11.20580236781278671287509496323764324188232421875;-19.6533310644436909342402941547334194183349609375;-9.7139589946325610725352817098610103130340576171875;7.19598103171827840895957706379704177379608154296875;2.17722867003912501360218811896629631519317626953125;0.491965854746570119271353860312956385314464569091796875;6.05841375062404541296245952253229916095733642578125;-5.27674362439168920246856941957958042621612548828125;0.2253522514789967345905097317881882190704345703125;2.90368687377947320982229939545504748821258544921875;10.839454844901805330437127850018441677093505859375;0.28456662512803887477019770813058130443096160888671875;7.220661017464994557712998357601463794708251953125;12.034435586999560285903498879633843898773193359375;11.4022395725051435277919154032133519649505615234375;-10.4812298521025102360226810560561716556549072265625;1.114420225544965337149960760143585503101348876953125;-18.999358449622004485490833758376538753509521484375;0.7990177471316239898868616364779882133007049560546875]
      mask Display: e = 0.06;c1 = [120 150 230]/255;c2 = ([120 150 230]+0)/383;c3 = ([120 150 230]+128)/383;patch([0 1 1 0],[0 0 1 1],c1);patch([0 1 1 1-e 1-e 0+e],[0 0 1 1-e 0+e 0+e],c2);patch([0 0 1 1-e 0+e 0+e],[0 1 1 1-e 1-e 0+e],c3);plot([0 1 1 0 0],[0 0 1 1 0]);disp('weights');
  Mux : Mux  Inputs=1
      mask Display: e = 0.06;c1 = [120 150 230]/255;c2 = ([120 150 230]+0)/383;c3 = ([120 150 230]+128)/383;patch([0 1 1 0],[0 0 1 1],c1);patch([0 1 1 1-e 1-e 0+e],[0 0 1 1-e 0+e 0+e],c2);patch([0 0 1 1-e 0+e 0+e],[0 1 1 1-e 1-e 0+e],c3);plot([0 1 1 0 0],[0 0 1 1 0]);disp('Mux');
  dotprod1 : neural/Weight Functions/dotprod
  "lz{2,1}" : Outport
      mask Display: e = 0.06;c1 = [120 230 180]/255;c2 = ([120 230 180]+0)/(256+128);c3 = ([120 230 180]+128)/(256+128);patch([0 1 1 0],[0 0 1 1],c1);patch([0 1 1 1-e 1-e 0+e],[0 0 1 1-e 0+e 0+e],c2);patch([0 0 1 1-e 0+e 0+e],[0 1 1 1-e 1-e 0+e],c3);plot([0 1 1 0 0],[0 0 1 1 0]);
  wires:
  Mux/1 -> "lz{2,1}"/1
  dotprod1/1 -> Mux/1
  "ad{2,1}"/1 -> dotprod1/2
  "IW{2,1}(1,:)'"/1 -> dotprod1/1

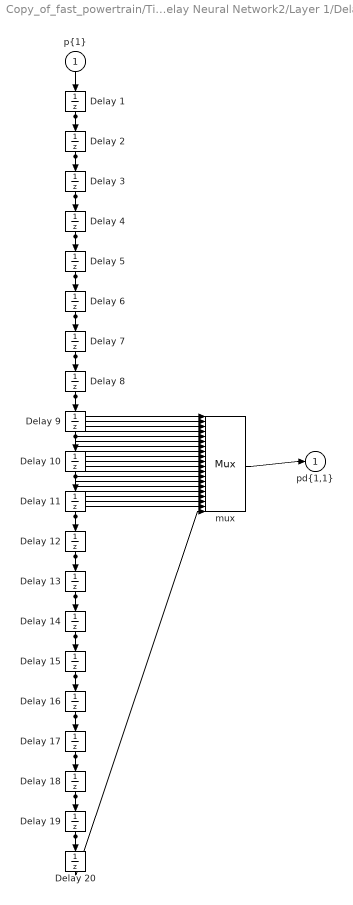
== system Copy_of_fast_powertrain/Time Delay Neural Network2/Layer 1/Delays 1 ==
  "p{1}" : Inport  PortDimensions=1  SampleTime=0.01
      mask Display: e = 0.06;c1 = [120 230 180]/255;c2 = ([120 230 180]+0)/(256+128);c3 = ([120 230 180]+128)/(256+128);patch([0 1 1 0],[0 0 1 1],c1);patch([0 1 1 1-e 1-e 0+e],[0 0 1 1-e 0+e 0+e],c2);patch([0 0 1 1-e 0+e 0+e],[0 1 1 1-e 1-e 0+e],c3);plot([0 1 1 0 0],[0 0 1 1 0]);
  Delay 1 : UnitDelay  InitialCondition=pi_input_1_delayed_1  SampleTime=0.01
      mask Display: e = 0.06;c1 = [120 150 230]/255;c2 = ([120 150 230]+0)/383;c3 = ([120 150 230]+128)/383;patch([0 1 1 0],[0 0 1 1],c1);patch([0 1 1 1-e 1-e 0+e],[0 0 1 1-e 0+e 0+e],c2);patch([0 0 1 1-e 0+e 0+e],[0 1 1 1-e 1-e 0+e],c3);plot([0 1 1 0 0],[0 0 1 1 0]);disp('D')
  Delay 10 : UnitDelay  InitialCondition=pi_input_1_delayed_10  SampleTime=0.01
      mask Display: e = 0.06;c1 = [120 150 230]/255;c2 = ([120 150 230]+0)/383;c3 = ([120 150 230]+128)/383;patch([0 1 1 0],[0 0 1 1],c1);patch([0 1 1 1-e 1-e 0+e],[0 0 1 1-e 0+e 0+e],c2);patch([0 0 1 1-e 0+e 0+e],[0 1 1 1-e 1-e 0+e],c3);plot([0 1 1 0 0],[0 0 1 1 0]);disp('D')
  Delay 11 : UnitDelay  InitialCondition=pi_input_1_delayed_11  SampleTime=0.01
      mask Display: e = 0.06;c1 = [120 150 230]/255;c2 = ([120 150 230]+0)/383;c3 = ([120 150 230]+128)/383;patch([0 1 1 0],[0 0 1 1],c1);patch([0 1 1 1-e 1-e 0+e],[0 0 1 1-e 0+e 0+e],c2);patch([0 0 1 1-e 0+e 0+e],[0 1 1 1-e 1-e 0+e],c3);plot([0 1 1 0 0],[0 0 1 1 0]);disp('D')
  Delay 12 : UnitDelay  InitialCondition=pi_input_1_delayed_12  SampleTime=0.01
      mask Display: e = 0.06;c1 = [120 150 230]/255;c2 = ([120 150 230]+0)/383;c3 = ([120 150 230]+128)/383;patch([0 1 1 0],[0 0 1 1],c1);patch([0 1 1 1-e 1-e 0+e],[0 0 1 1-e 0+e 0+e],c2);patch([0 0 1 1-e 0+e 0+e],[0 1 1 1-e 1-e 0+e],c3);plot([0 1 1 0 0],[0 0 1 1 0]);disp('D')
  Delay 13 : UnitDelay  InitialCondition=pi_input_1_delayed_13  SampleTime=0.01
      mask Display: e = 0.06;c1 = [120 150 230]/255;c2 = ([120 150 230]+0)/383;c3 = ([120 150 230]+128)/383;patch([0 1 1 0],[0 0 1 1],c1);patch([0 1 1 1-e 1-e 0+e],[0 0 1 1-e 0+e 0+e],c2);patch([0 0 1 1-e 0+e 0+e],[0 1 1 1-e 1-e 0+e],c3);plot([0 1 1 0 0],[0 0 1 1 0]);disp('D')
  Delay 14 : UnitDelay  InitialCondition=pi_input_1_delayed_14  SampleTime=0.01
      mask Display: e = 0.06;c1 = [120 150 230]/255;c2 = ([120 150 230]+0)/383;c3 = ([120 150 230]+128)/383;patch([0 1 1 0],[0 0 1 1],c1);patch([0 1 1 1-e 1-e 0+e],[0 0 1 1-e 0+e 0+e],c2);patch([0 0 1 1-e 0+e 0+e],[0 1 1 1-e 1-e 0+e],c3);plot([0 1 1 0 0],[0 0 1 1 0]);disp('D')
  Delay 15 : UnitDelay  InitialCondition=pi_input_1_delayed_15  SampleTime=0.01
      mask Display: e = 0.06;c1 = [120 150 230]/255;c2 = ([120 150 230]+0)/383;c3 = ([120 150 230]+128)/383;patch([0 1 1 0],[0 0 1 1],c1);patch([0 1 1 1-e 1-e 0+e],[0 0 1 1-e 0+e 0+e],c2);patch([0 0 1 1-e 0+e 0+e],[0 1 1 1-e 1-e 0+e],c3);plot([0 1 1 0 0],[0 0 1 1 0]);disp('D')
  Delay 16 : UnitDelay  InitialCondition=pi_input_1_delayed_16  SampleTime=0.01
      mask Display: e = 0.06;c1 = [120 150 230]/255;c2 = ([120 150 230]+0)/383;c3 = ([120 150 230]+128)/383;patch([0 1 1 0],[0 0 1 1],c1);patch([0 1 1 1-e 1-e 0+e],[0 0 1 1-e 0+e 0+e],c2);patch([0 0 1 1-e 0+e 0+e],[0 1 1 1-e 1-e 0+e],c3);plot([0 1 1 0 0],[0 0 1 1 0]);disp('D')
  Delay 17 : UnitDelay  InitialCondition=pi_input_1_delayed_17  SampleTime=0.01
      mask Display: e = 0.06;c1 = [120 150 230]/255;c2 = ([120 150 230]+0)/383;c3 = ([120 150 230]+128)/383;patch([0 1 1 0],[0 0 1 1],c1);patch([0 1 1 1-e 1-e 0+e],[0 0 1 1-e 0+e 0+e],c2);patch([0 0 1 1-e 0+e 0+e],[0 1 1 1-e 1-e 0+e],c3);plot([0 1 1 0 0],[0 0 1 1 0]);disp('D')
  Delay 18 : UnitDelay  InitialCondition=pi_input_1_delayed_18  SampleTime=0.01
      mask Display: e = 0.06;c1 = [120 150 230]/255;c2 = ([120 150 230]+0)/383;c3 = ([120 150 230]+128)/383;patch([0 1 1 0],[0 0 1 1],c1);patch([0 1 1 1-e 1-e 0+e],[0 0 1 1-e 0+e 0+e],c2);patch([0 0 1 1-e 0+e 0+e],[0 1 1 1-e 1-e 0+e],c3);plot([0 1 1 0 0],[0 0 1 1 0]);disp('D')
  Delay 19 : UnitDelay  InitialCondition=pi_input_1_delayed_19  SampleTime=0.01
      mask Display: e = 0.06;c1 = [120 150 230]/255;c2 = ([120 150 230]+0)/383;c3 = ([120 150 230]+128)/383;patch([0 1 1 0],[0 0 1 1],c1);patch([0 1 1 1-e 1-e 0+e],[0 0 1 1-e 0+e 0+e],c2);patch([0 0 1 1-e 0+e 0+e],[0 1 1 1-e 1-e 0+e],c3);plot([0 1 1 0 0],[0 0 1 1 0]);disp('D')
  Delay 2 : UnitDelay  InitialCondition=pi_input_1_delayed_2  SampleTime=0.01
      mask Display: e = 0.06;c1 = [120 150 230]/255;c2 = ([120 150 230]+0)/383;c3 = ([120 150 230]+128)/383;patch([0 1 1 0],[0 0 1 1],c1);patch([0 1 1 1-e 1-e 0+e],[0 0 1 1-e 0+e 0+e],c2);patch([0 0 1 1-e 0+e 0+e],[0 1 1 1-e 1-e 0+e],c3);plot([0 1 1 0 0],[0 0 1 1 0]);disp('D')
  Delay 20 : UnitDelay  InitialCondition=pi_input_1_delayed_20  SampleTime=0.01
      mask Display: e = 0.06;c1 = [120 150 230]/255;c2 = ([120 150 230]+0)/383;c3 = ([120 150 230]+128)/383;patch([0 1 1 0],[0 0 1 1],c1);patch([0 1 1 1-e 1-e 0+e],[0 0 1 1-e 0+e 0+e],c2);patch([0 0 1 1-e 0+e 0+e],[0 1 1 1-e 1-e 0+e],c3);plot([0 1 1 0 0],[0 0 1 1 0]);disp('D')
  Delay 3 : UnitDelay  InitialCondition=pi_input_1_delayed_3  SampleTime=0.01
      mask Display: e = 0.06;c1 = [120 150 230]/255;c2 = ([120 150 230]+0)/383;c3 = ([120 150 230]+128)/383;patch([0 1 1 0],[0 0 1 1],c1);patch([0 1 1 1-e 1-e 0+e],[0 0 1 1-e 0+e 0+e],c2);patch([0 0 1 1-e 0+e 0+e],[0 1 1 1-e 1-e 0+e],c3);plot([0 1 1 0 0],[0 0 1 1 0]);disp('D')
  Delay 4 : UnitDelay  InitialCondition=pi_input_1_delayed_4  SampleTime=0.01
      mask Display: e = 0.06;c1 = [120 150 230]/255;c2 = ([120 150 230]+0)/383;c3 = ([120 150 230]+128)/383;patch([0 1 1 0],[0 0 1 1],c1);patch([0 1 1 1-e 1-e 0+e],[0 0 1 1-e 0+e 0+e],c2);patch([0 0 1 1-e 0+e 0+e],[0 1 1 1-e 1-e 0+e],c3);plot([0 1 1 0 0],[0 0 1 1 0]);disp('D')
  Delay 5 : UnitDelay  InitialCondition=pi_input_1_delayed_5  SampleTime=0.01
      mask Display: e = 0.06;c1 = [120 150 230]/255;c2 = ([120 150 230]+0)/383;c3 = ([120 150 230]+128)/383;patch([0 1 1 0],[0 0 1 1],c1);patch([0 1 1 1-e 1-e 0+e],[0 0 1 1-e 0+e 0+e],c2);patch([0 0 1 1-e 0+e 0+e],[0 1 1 1-e 1-e 0+e],c3);plot([0 1 1 0 0],[0 0 1 1 0]);disp('D')
  Delay 6 : UnitDelay  InitialCondition=pi_input_1_delayed_6  SampleTime=0.01
      mask Display: e = 0.06;c1 = [120 150 230]/255;c2 = ([120 150 230]+0)/383;c3 = ([120 150 230]+128)/383;patch([0 1 1 0],[0 0 1 1],c1);patch([0 1 1 1-e 1-e 0+e],[0 0 1 1-e 0+e 0+e],c2);patch([0 0 1 1-e 0+e 0+e],[0 1 1 1-e 1-e 0+e],c3);plot([0 1 1 0 0],[0 0 1 1 0]);disp('D')
  Delay 7 : UnitDelay  InitialCondition=pi_input_1_delayed_7  SampleTime=0.01
      mask Display: e = 0.06;c1 = [120 150 230]/255;c2 = ([120 150 230]+0)/383;c3 = ([120 150 230]+128)/383;patch([0 1 1 0],[0 0 1 1],c1);patch([0 1 1 1-e 1-e 0+e],[0 0 1 1-e 0+e 0+e],c2);patch([0 0 1 1-e 0+e 0+e],[0 1 1 1-e 1-e 0+e],c3);plot([0 1 1 0 0],[0 0 1 1 0]);disp('D')
  Delay 8 : UnitDelay  InitialCondition=pi_input_1_delayed_8  SampleTime=0.01
      mask Display: e = 0.06;c1 = [120 150 230]/255;c2 = ([120 150 230]+0)/383;c3 = ([120 150 230]+128)/383;patch([0 1 1 0],[0 0 1 1],c1);patch([0 1 1 1-e 1-e 0+e],[0 0 1 1-e 0+e 0+e],c2);patch([0 0 1 1-e 0+e 0+e],[0 1 1 1-e 1-e 0+e],c3);plot([0 1 1 0 0],[0 0 1 1 0]);disp('D')
  Delay 9 : UnitDelay  InitialCondition=pi_input_1_delayed_9  SampleTime=0.01
      mask Display: e = 0.06;c1 = [120 150 230]/255;c2 = ([120 150 230]+0)/383;c3 = ([120 150 230]+128)/383;patch([0 1 1 0],[0 0 1 1],c1);patch([0 1 1 1-e 1-e 0+e],[0 0 1 1-e 0+e 0+e],c2);patch([0 0 1 1-e 0+e 0+e],[0 1 1 1-e 1-e 0+e],c3);plot([0 1 1 0 0],[0 0 1 1 0]);disp('D')
  mux : Mux  Inputs=20
      mask Display: e = 0.06;c1 = [120 150 230]/255;c2 = ([120 150 230]+0)/383;c3 = ([120 150 230]+128)/383;patch([0 1 1 0],[0 0 1 1],c1);patch([0 1 1 1-e 1-e 0+e],[0 0 1 1-e 0+e 0+e],c2);patch([0 0 1 1-e 0+e 0+e],[0 1 1 1-e 1-e 0+e],c3);plot([0 1 1 0 0],[0 0 1 1 0]);disp('Mux')
  "pd{1,1}" : Outport
      mask Display: e = 0.06;c1 = [120 230 180]/255;c2 = ([120 230 180]+0)/(256+128);c3 = ([120 230 180]+128)/(256+128);patch([0 1 1 0],[0 0 1 1],c1);patch([0 1 1 1-e 1-e 0+e],[0 0 1 1-e 0+e 0+e],c2);patch([0 0 1 1-e 0+e 0+e],[0 1 1 1-e 1-e 0+e],c3);plot([0 1 1 0 0],[0 0 1 1 0]);
  wires:
  mux/1 -> "pd{1,1}"/1
  Delay 20/1 -> mux/20
  Delay 19/1 -> mux/19, Delay 20/1
  Delay 18/1 -> mux/18, Delay 19/1
  Delay 17/1 -> mux/17, Delay 18/1
  Delay 16/1 -> mux/16, Delay 17/1
  Delay 15/1 -> mux/15, Delay 16/1
  Delay 14/1 -> mux/14, Delay 15/1
  Delay 13/1 -> mux/13, Delay 14/1
  Delay 12/1 -> mux/12, Delay 13/1
  Delay 11/1 -> mux/11, Delay 12/1
  Delay 10/1 -> mux/10, Delay 11/1
  Delay 9/1 -> mux/9, Delay 10/1
  Delay 8/1 -> mux/8, Delay 9/1
  Delay 7/1 -> mux/7, Delay 8/1
  Delay 6/1 -> mux/6, Delay 7/1
  Delay 5/1 -> mux/5, Delay 6/1
  Delay 4/1 -> mux/4, Delay 5/1
  Delay 3/1 -> mux/3, Delay 4/1
  Delay 2/1 -> mux/2, Delay 3/1
  Delay 1/1 -> mux/1, Delay 2/1
  "p{1}"/1 -> Delay 1/1
